simulink model "Problem_No10"  (R2020a)
settings: Solver=VariableStepAuto  StartTime=0.0  StopTime=10.0  RelTol=1e-3
libraries: simulink x1
settings Model: Creator='Z'ome  LastModifiedBy=Animesh Uttekar

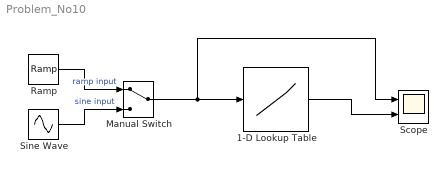
== system Problem_No10 ==
  1-D Lookup Table : Lookup_n-D  NumberOfTableDimensions=1  BreakpointsForDimension1=[0.000 0.072 0.198 0.290 0.426 0.511 0.543 0.573 0.600 0.610 0.628 0.640 0.651 0.662 0.672 0.680 0.691 0.697 0.703 0.710 0.712]  Table=[0.00 0.00 0.00 0.00 0.03 0.22 0.44 0.85 1.50 1.87 2.76 3.57 4.48 5.69 7.11 8.44 10.86 12.73 14.24 16.91 17.63]  InternalRulePriority=Speed  RndMeth=Simplest  InputSameDT=on
  Manual Switch : ManualSwitch
  Ramp : simulink/Sources/Ramp  slope=1  start=0  InitialOutput=0
  Scope : Scope  NumInputPorts=2
  Sine Wave : Sin  SampleTime=0
  wires:
  1-D Lookup Table/1 -> Scope/2
  Manual Switch/1 -> 1-D Lookup Table/1, Scope/1
  Sine Wave/1 -> Manual Switch/2  "sine input"
  Ramp/1 -> Manual Switch/1  "ramp input"
